simulink model "sldemo_mdlref_variants"  (Simulink 7.6)
settings: Solver=FixedStepDiscrete  StartTime=0.0  StopTime=10.0  RelTol=1e-3
PreLoadFcn:
  | V_NONLINEAR_CONTROLLER=Simulink.Variant('CTRL==1')
  | V_SECOND_ORDER_CONTROLLER=Simulink.Variant('CTRL==2')
  | 
  | CTRL=1
Description:
  | Model Reference Variants
  | 
  | This demo illustrates model reference variants. A Model block is used to
  | reference one Simulink(R) model from another Simulink model. A Model block can
  | have different variants. A variant describes one of N possible modes a Model
  | block can operate in. Each variant of the Model block references a specific
  | model with model specific arguments. Only one variant is active for
  | simulation. You can switch the active variant of a Model block by changing the
  | values of variables in the base workspace or manually overriding variant
  | selection using the Model block dialog.
settings Model: Creator=The MathWorks Inc.
settings OptimizationCC: InlineParams=on
settings RTWCC: ProcessScript=grt_make_rtw_hook

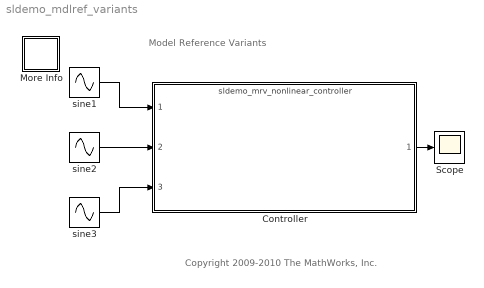
== system sldemo_mdlref_variants ==
  note: Copyright 2009-2010 The MathWorks, Inc.
  note: Model Reference Variants
  Controller : ModelReference  ModelNameDialog=sldemo_mrv_nonlinear_controller  SimulationMode=Normal  Variant=on  ModelReferenceVersion=1.9  CopyOfModelName=sldemo_mrv_nonlinear_controller
      settings: AttributesFormatString=%<ActiveVariant>  GeneratePreprocessorConditionals=on
  More Info : Subsystem
      settings: OpenFcn=showdemo(bdroot(gcb))
      mask Display: disp('?')
  Scope : Scope
  sine1 : Sin  Amplitude=.1  Frequency=pi/3  SampleTime=.01
  sine2 : Sin  Amplitude=2  SampleTime=.01
  sine3 : Sin  Amplitude=.3  Frequency=pi/6  SampleTime=.01
  wires:
  sine2/1 -> Controller/2
  sine1/1 -> Controller/1
  sine3/1 -> Controller/3
  Controller/1 -> Scope/1

== system sldemo_mdlref_variants/More Info ==
  note: This demo illustrates model reference variants. A Model block is used to
      | reference one Simulink model from another Simulink model. A Model block can
      | have different variants. A variant describes one of N possible modes a Model
      | block can operate in. Each variant of the Model block references a specific
      | model with model specific arguments. Only one variant is active for
      | simulation. You can switch the active variant of a Model block by changing the
      | values of variables in the base workspace or manually overriding variant
      | selection using the Model block dialog.
  note: Model Reference Variants
